simulink model "buoi2_DSB_FC"  (R2020b)
settings: Solver=VariableStepAuto  StartTime=0.0  StopTime=10.0  RelTol=1e-3
libraries: dsparch4 x1
settings Model: Creator=htn  LastModifiedBy=htn

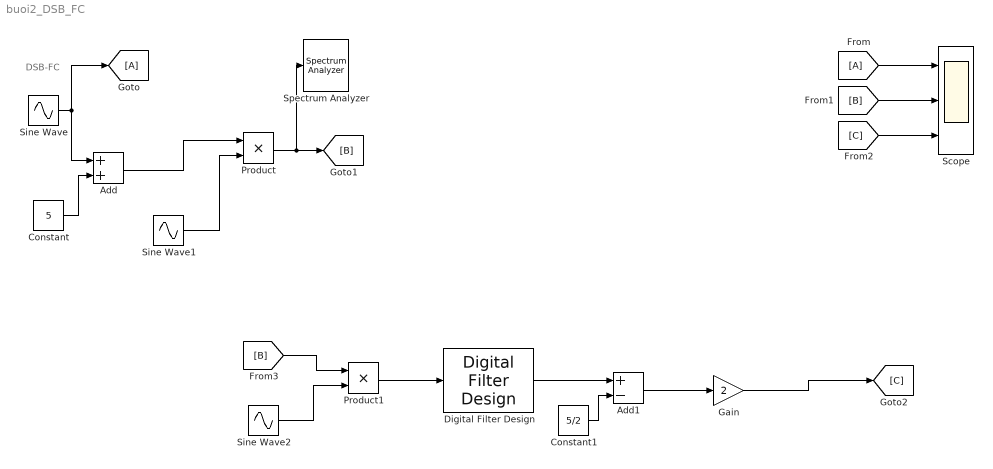
== system buoi2_DSB_FC ==
  note: DSB-FC
  Add : Sum
  Add1 : Sum  Inputs=+-
  Constant : Constant  Value=5
  Constant1 : Constant  Value=5/2
  Digital Filter Design : dsparch4/Digital Filter Design  mwdsp_browser_bugfix_var=off
  Gain : Gain  Gain=2
  Product : Product
  Product1 : Product
  Scope : Scope  NumInputPorts=3
  Sine Wave : Sin  Frequency=2*pi*200  SampleTime=1/50000
  Sine Wave1 : Sin  Frequency=2*pi*5000  SampleTime=1/50000
  Sine Wave2 : Sin  Frequency=2*pi*5000  SampleTime=1/50000
  Spectrum Analyzer : SpectrumAnalyzer
  wires:
  Constant/1 -> Add/2
  Sine Wave/1 -> [A], Add/1
  Add/1 -> Product/1
  Sine Wave1/1 -> Product/2
  [A] -> Scope/1
  [B] -> Scope/2
  [C] -> Scope/3
  Product/1 -> Spectrum Analyzer/1, [B]
  Sine Wave2/1 -> Product1/2
  [B] -> Product1/1
  Product1/1 -> Digital Filter Design/1
  Digital Filter Design/1 -> Add1/1
  Constant1/1 -> Add1/2
  Add1/1 -> Gain/1
  Gain/1 -> [C]
